simulink model "Figure_2_3_TP_Telecom_modulation_demodulation_ASK2"  (R2020a)
settings: Solver=VariableStepAuto  StartTime=0.0  StopTime=20  RelTol=1e-3
libraries: commutil2 x6, dspsigops x4, dspsrcs4 x4, simulink x2, commrandsrc3 x2, commsink2 x1
settings Model: Creator=iba  LastModifiedBy=iba

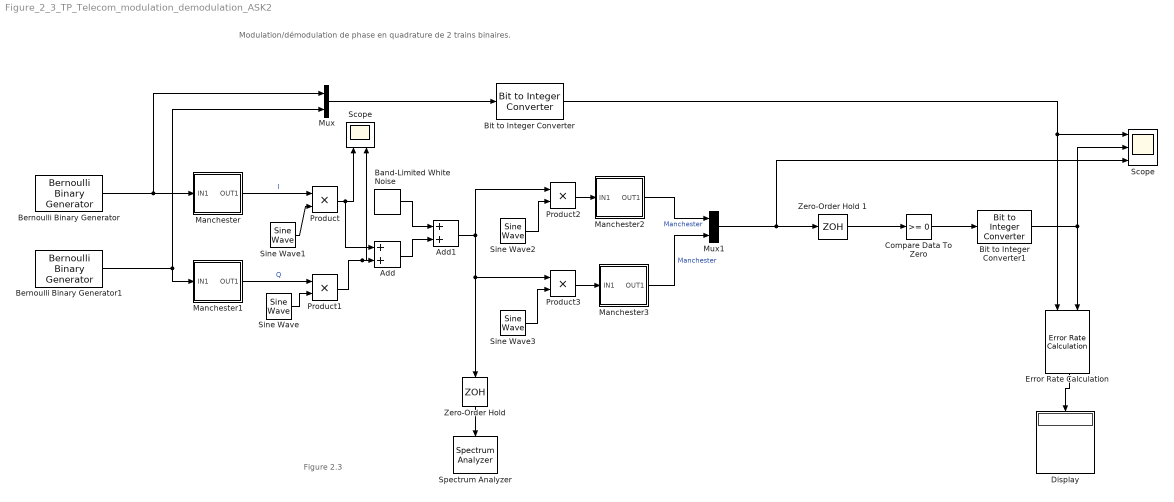
== system Figure_2_3_TP_Telecom_modulation_demodulation_ASK2 ==
  note: Figure 2.3
  note: Modulation/démodulation de phase en quadrature de 2 trains binaires.
  Add : Sum
  Add1 : Sum
  Band-Limited White Noise : simulink/Sources/Band-Limited White Noise  Cov=[1e-3]  Ts=0.1  seed=[23341]
  Bernoulli Binary Generator : commrandsrc3/Bernoulli Binary Generator  ProbabilityOfZero=0.5  SeedSource=Parameter  Seed=32  SampleTime=1  SamplesPerFrame=1  OutputDataType=double  SimulateUsing=Interpreted execution
  Bernoulli Binary Generator1 : commrandsrc3/Bernoulli Binary Generator  ProbabilityOfZero=0.5  SeedSource=Parameter  Seed=24  SampleTime=1  SamplesPerFrame=1  OutputDataType=double  SimulateUsing=Interpreted execution
  Bit to Integer Converter : commutil2/Bit to Integer Converter  nbits=2  bitOrder=MSB first  signedOutputValues=Unsigned  outDtype=Inherit via internal rule  outDtypeSigned=Inherit via internal rule
  "Bit to Integer Converter1 " : commutil2/Bit to Integer Converter  nbits=8  bitOrder=MSB first  signedOutputValues=Unsigned  outDtype=double  outDtypeSigned=Inherit via internal rule
  Compare Data To Zero : simulink/Logic and Bit Operations/Compare To Zero  relop=>=  OutDataTypeStr=uint8
  "Display " : Display
  Error Rate Calculation : commsink2/Error Rate Calculation  N=0  st_delay=0  cp_mode=Entire frame  subframe=[]  PMode=Port  WsName=ErrorVec  RsMode2=off  stop=on  numErr=100  maxBits=100
  Manchester : Subsystem
  Manchester1 : Subsystem
  Manchester2 : Subsystem
  Manchester3 : Subsystem
  Mux : Mux  Inputs=2
  Mux1 : Mux  Inputs=2
  "Product " : Product
  "Product1 " : Product
  Product2 : Product
  Product3 : Product
  Scope : Scope  NumInputPorts=2
  "Scope " : Scope  NumInputPorts=3
  Sine Wave : dspsrcs4/Sine Wave  Amplitude=1  Frequency=5  Phase=0  SampleMode=Discrete  OutComplex=Real  CompMethod=Trigonometric fcn  TableSize=Speed  SampleTime=1/100  SamplesPerFrame=1  ResetState=Restart at time zero  OutputFrames=off  dataType=double  wordLen=16  udDataType=sfix(16)  fracBitsMode=Best precision  numFracBits=15  OutDataTypeStr=double  LastOutDataTypeStr=double
  Sine Wave1 : dspsrcs4/Sine Wave  Amplitude=1  Frequency=5  Phase=pi/2  SampleMode=Discrete  OutComplex=Real  CompMethod=Trigonometric fcn  TableSize=Speed  SampleTime=1/100  SamplesPerFrame=1  ResetState=Restart at time zero  OutputFrames=off  dataType=double  wordLen=16  udDataType=sfix(16)  fracBitsMode=Best precision  numFracBits=15  OutDataTypeStr=double  LastOutDataTypeStr=double
  Sine Wave2 : dspsrcs4/Sine Wave  Amplitude=1  Frequency=5  Phase=pi/2  SampleMode=Discrete  OutComplex=Real  CompMethod=Trigonometric fcn  TableSize=Speed  SampleTime=1  SamplesPerFrame=1  ResetState=Restart at time zero  OutputFrames=off  dataType=double  wordLen=16  udDataType=sfix(16)  fracBitsMode=Best precision  numFracBits=15  OutDataTypeStr=double  LastOutDataTypeStr=double
  Sine Wave3 : dspsrcs4/Sine Wave  Amplitude=1  Frequency=5  Phase=0  SampleMode=Discrete  OutComplex=Real  CompMethod=Trigonometric fcn  TableSize=Speed  SampleTime=1  SamplesPerFrame=1  ResetState=Restart at time zero  OutputFrames=off  dataType=double  wordLen=16  udDataType=sfix(16)  fracBitsMode=Best precision  numFracBits=15  OutDataTypeStr=double  LastOutDataTypeStr=double
  Spectrum Analyzer : SpectrumAnalyzer
  "Zero-Order Hold " : ZeroOrderHold  SampleTime=-1
  Zero-Order Hold 1 : ZeroOrderHold
  wires:
  Bernoulli Binary Generator/1 -> Manchester/1(IN1), Mux/1
  Bernoulli Binary Generator1/1 -> Mux/2, Manchester1/1(IN1)
  "Product "/1 -> Add/1, Scope/1
  Sine Wave/1 -> "Product1 "/2
  Sine Wave1/1 -> "Product "/2
  "Product1 "/1 -> Scope/2, Add/2
  Mux/1 -> Bit to Integer Converter/1
  Bit to Integer Converter/1 -> Error Rate Calculation/1, "Scope "/1
  "Bit to Integer Converter1 "/1 -> "Scope "/2, Error Rate Calculation/2
  Mux1/1 -> "Scope "/3, Zero-Order Hold 1/1
  Sine Wave3/1 -> Product3/2
  Sine Wave2/1 -> Product2/2
  Add/1 -> Add1/2
  "Zero-Order Hold "/1 -> Spectrum Analyzer/1
  Band-Limited White Noise/1 -> Add1/1
  Add1/1 -> Product3/1, "Zero-Order Hold "/1, Product2/1
  Error Rate Calculation/1 -> "Display "/1
  Manchester/1(OUT1) -> "Product "/1  "I"
  Manchester1/1(OUT1) -> "Product1 "/1  "Q"
  Product2/1 -> Manchester2/1(IN1)
  Product3/1 -> Manchester3/1(IN1)
  Manchester3/1(OUT1) -> Mux1/2  "Manchester"
  Manchester2/1(OUT1) -> Mux1/1  "Manchester"
  Zero-Order Hold 1/1 -> Compare Data To Zero/1
  Compare Data To Zero/1 -> "Bit to Integer Converter1 "/1

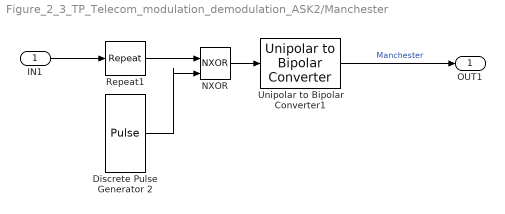
== system Figure_2_3_TP_Telecom_modulation_demodulation_ASK2/Manchester ==
  IN1 : Inport
  "Discrete Pulse Generator 2  " : DiscretePulseGenerator  SampleTime=0.01
  "NXOR " : Logic  Operator=NXOR  IconShape=distinctive  AllPortsSameDT=off  OutDataTypeStr=boolean
  Repeat1 : dspsigops/Repeat  N=2  InputProcessing=Columns as channels (frame based)  RateOptions=Enforce single-rate processing  ic=0  mode=Unused parameter value
  Unipolar to Bipolar Converter1 : commutil2/Unipolar to Bipolar Converter  M=2  polarity=Positive  dataType=double
  OUT1 : Outport
  wires:
  IN1/1 -> Repeat1/1
  "NXOR "/1 -> Unipolar to Bipolar Converter1/1
  "Discrete Pulse Generator 2  "/1 -> "NXOR "/2
  Unipolar to Bipolar Converter1/1 -> OUT1/1  "Manchester"
  Repeat1/1 -> "NXOR "/1

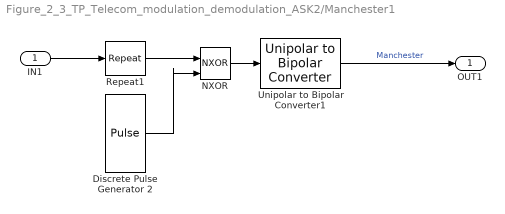
== system Figure_2_3_TP_Telecom_modulation_demodulation_ASK2/Manchester1 ==
  IN1 : Inport
  "Discrete Pulse Generator 2  " : DiscretePulseGenerator  SampleTime=0.5
  "NXOR " : Logic  Operator=NXOR  IconShape=distinctive  AllPortsSameDT=off  OutDataTypeStr=boolean
  Repeat1 : dspsigops/Repeat  N=2  InputProcessing=Columns as channels (frame based)  RateOptions=Enforce single-rate processing  ic=0  mode=Unused parameter value
  Unipolar to Bipolar Converter1 : commutil2/Unipolar to Bipolar Converter  M=2  polarity=Positive  dataType=double
  OUT1 : Outport
  wires:
  Repeat1/1 -> "NXOR "/1
  Unipolar to Bipolar Converter1/1 -> OUT1/1  "Manchester"
  "Discrete Pulse Generator 2  "/1 -> "NXOR "/2
  "NXOR "/1 -> Unipolar to Bipolar Converter1/1
  IN1/1 -> Repeat1/1

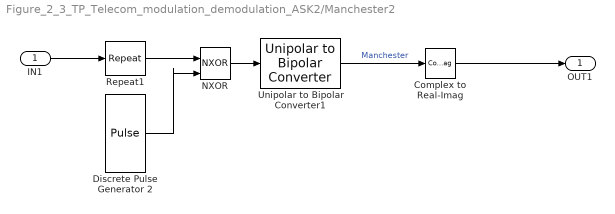
== system Figure_2_3_TP_Telecom_modulation_demodulation_ASK2/Manchester2 ==
  IN1 : Inport
  Complex to Real-Imag : ComplexToRealImag  Output=Imag
  "Discrete Pulse Generator 2  " : DiscretePulseGenerator  SampleTime=0.5
  "NXOR " : Logic  Operator=NXOR  IconShape=distinctive  AllPortsSameDT=off  OutDataTypeStr=boolean
  Repeat1 : dspsigops/Repeat  N=2  InputProcessing=Columns as channels (frame based)  RateOptions=Enforce single-rate processing  ic=0  mode=Unused parameter value
  Unipolar to Bipolar Converter1 : commutil2/Unipolar to Bipolar Converter  M=2  polarity=Positive  dataType=double
  OUT1 : Outport
  wires:
  IN1/1 -> Repeat1/1
  "NXOR "/1 -> Unipolar to Bipolar Converter1/1
  "Discrete Pulse Generator 2  "/1 -> "NXOR "/2
  Repeat1/1 -> "NXOR "/1
  Unipolar to Bipolar Converter1/1 -> Complex to Real-Imag/1  "Manchester"
  Complex to Real-Imag/1 -> OUT1/1

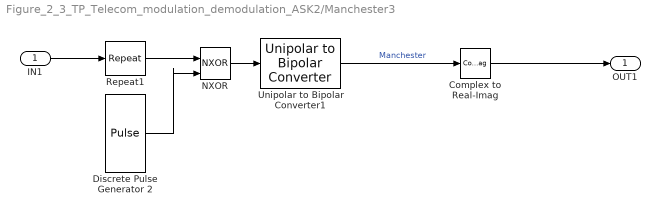
== system Figure_2_3_TP_Telecom_modulation_demodulation_ASK2/Manchester3 ==
  IN1 : Inport
  Complex to Real-Imag : ComplexToRealImag  Output=Real
  "Discrete Pulse Generator 2  " : DiscretePulseGenerator  SampleTime=0.5
  "NXOR " : Logic  Operator=NXOR  IconShape=distinctive  AllPortsSameDT=off  OutDataTypeStr=boolean
  Repeat1 : dspsigops/Repeat  N=2  InputProcessing=Columns as channels (frame based)  RateOptions=Enforce single-rate processing  ic=0  mode=Unused parameter value
  Unipolar to Bipolar Converter1 : commutil2/Unipolar to Bipolar Converter  M=2  polarity=Positive  dataType=double
  OUT1 : Outport
  wires:
  Repeat1/1 -> "NXOR "/1
  "Discrete Pulse Generator 2  "/1 -> "NXOR "/2
  "NXOR "/1 -> Unipolar to Bipolar Converter1/1
  IN1/1 -> Repeat1/1
  Unipolar to Bipolar Converter1/1 -> Complex to Real-Imag/1  "Manchester"
  Complex to Real-Imag/1 -> OUT1/1
